simulink model "QuadrotorModel"  (R2023b)
settings: Solver=VariableStepAuto  StartTime=0.0  StopTime=120  RelTol=1e-3
undefined symbols (not defined in the file): A, a1, a2, a3, a4, a5, B, b1, b2, b3, belokan, C, c1, c2, c3, c4, c5, c6, c7, c8, D, g, k1, k2, k3, k4, kecepatan, kf, km, lebar, m, OM_r, panjang, phi_dot_d, psi_dot_d, theta_dot_d, U1, U1_max, U2, U2_max, U3, U4, U4_max, z_dot_d
libraries: simulink_extras x6, sldrtlib x1
settings Model: Creator=izmah  LastModifiedBy=izmah
settings SolverCC: ZeroCrossAlgorithm=Adaptive
settings DebuggingCC: IgnoredZcDiagnostic=none

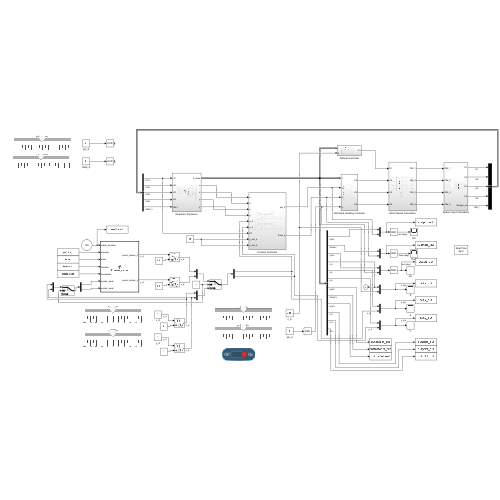
[thumbnail: Simulink's stored preview of the top-level diagram]
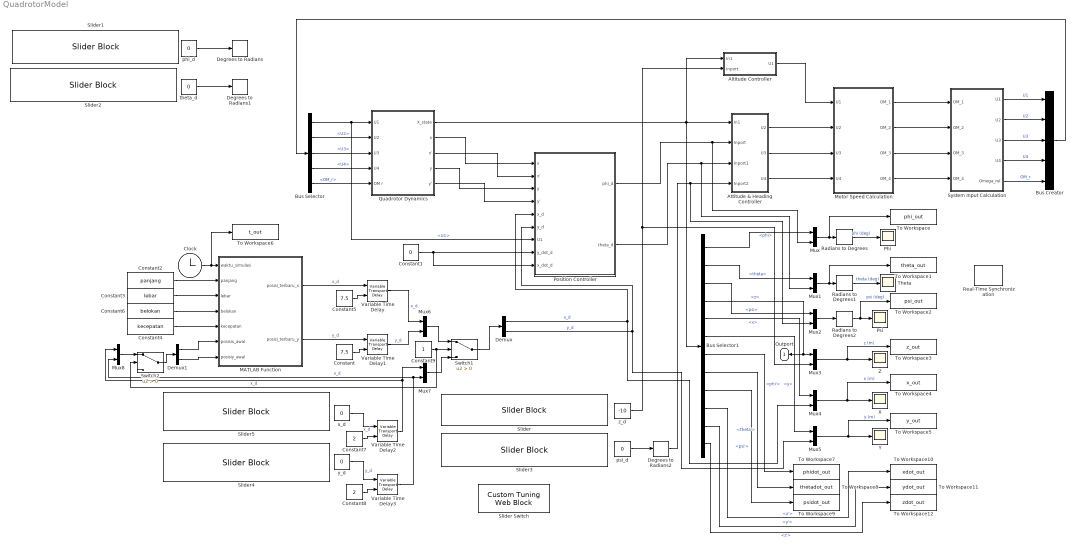
== system QuadrotorModel ==
  Altitude Controller : Subsystem
  Attitude & Heading Controller : Subsystem
  Bus Creator : BusCreator  Inputs=U1,U2,U3,U4,OM_r
  Bus Selector : BusSelector  OutputSignals=U1,U2,U3,U4,OM_r
  Bus Selector1 : BusSelector  OutputSignals=phi,theta,psi,z,x,y,phi',theta',psi',x',y',z'
  Clock : Clock
      settings: Decimation=waktu_simulasi
  Constant : Constant  Value=7.5
  Constant1 : Constant  Value=0
  Constant2 : Constant  Value=panjang
  Constant3 : Constant  Value=lebar
  Constant4 : Constant  Value=kecepatan
  Constant5 : Constant  Value=7.5
  Constant6 : Constant  Value=belokan
  Constant7 : Constant  Value=2
  Constant8 : Constant  Value=2
  Constant9 : Constant
  Degrees to Radians : simulink_extras/Transformations/Degrees to Radians
  Degrees to Radians1 : simulink_extras/Transformations/Degrees to Radians
  Degrees to Radians2 : simulink_extras/Transformations/Degrees to Radians
  Demux : Demux  Outputs=2
  Demux1 : Demux  Outputs=2
  MATLAB Function : MATLAB Function  TreatAsAtomicUnit=on
  Motor Speed Calculation : Subsystem
  Mux{,1..8} (9 alike) : Mux  Inputs=2
  Phi : Scope
  Position Controller : Subsystem
  Psi : Scope
  Quadrotor Dynamics : Subsystem
  Radians to Degrees : simulink_extras/Transformations/Radians to Degrees
  Radians to Degrees1 : simulink_extras/Transformations/Radians to Degrees
  Radians to Degrees2 : simulink_extras/Transformations/Radians to Degrees
  Real-Time Synchronization : sldrtlib/Real-Time Synchronization  SampleTime=0.1  MaxMissedTicks=1000  ShowMissedTicks=off  YieldWhenWaiting=off
  Slider : SliderBlock  ScaleMin=-20  ScaleMax=0
  Slider Switch : CustomTuningWebBlock  LabelPosition=Hide  ShowInitialText=on  Configuration="{\"components\":[{\"name\":\"CustomSwitchStateComponent\",\"settings\":{\"position\":[0,0,1,1],\"states\":[{\"HitRegion\":{\"position\":[0,0,0.5,1]},\"Image\":{\"position\":[0,0,1,1],\"size\":[1,1],\"src\":\"data:image\\/svg+xml;base64,PD94bWwgdmVyc2lvbj0iMS4wIiBlbmNvZGluZz0idXRmLTgiPz4NCjwhLS0gR2VuZXJhdG9yOiBBZG9iZSBJbGx1c3RyYXRvciAyNS4yLjEsIFNWRyBFeHBvcnQgUGx1Zy1JbiAuIFNWRyBWZXJzaW9uOiA2LjAwIEJ1aWxkIDApICAtLT4NCjxzdmcgdmVyc2lvbj0iMS4xIiB4bWxucz0iaHR0cDovL3d3dy53My5vcmcvMjAwMC9zdmciIHhtbG5zOnhsaW5rPSJodHRwOi8vd3d3LnczLm9yZy8xOTk5L3hsaW5rIiB4PSIwcHgiIHk9IjBweCINCgkgdmlld0JveD0iMCAwIDc2IDI5IiBzdHlsZT0iZW5hYmxlLWJhY2tncm91bmQ6bmV3 ...(+5404 chars)\",\"srcOrientation\":\"Right\"},\"Label\":{\"color\":[0.9882352941176471,0.9882352941176471,0.7725490196078432],\"icon\":{\"size\":[0,0],\"src\":[],\"srcOrientation\":\"Right\"},\"iconPlacement\":\"left\",\"opacity\":1,\"position\":[0.5,0.14],\"show\":true,\"text\":{\"content\":\"Off\",\"font\":\"Helvetica\",\"fontSize\":8.4}},\"Value\":-1},{\"HitRegion\":{\"position\":[0,0.5,0.5,1]},\"Image\":{\"position\":[0,0,1,1],\"size\":[1,1],\"src\":\"data:image\\/svg+xml;base64,PD94bWwgdmVyc2lvbj0iMS4wIiBlbmNvZGluZz0idXRmLTgiPz4NCjwhLS0gR2VuZXJhdG9yOiBBZG9iZSBJbGx1c3RyYXRvciAyNS4yLjEsIFNWRyBFeHBvcnQgUGx1Zy1JbiAuIFNWRyBWZXJzaW9uOiA2LjAwIEJ1aWxkIDApICAtLT4NCjxzdmcgdmVyc2lvbj0iMS4xIiB4bWxucz0iaHR0cDovL3d3dy53My5vcmcvMjAwMC9zdmciIHhtbG5zOnhsaW5rPSJodHRwOi8vd3d3LnczLm9yZy8xOTk5L3hsaW5rIiB4PSIwcHgiIHk9IjBweCINCgkgdmlld0JveD0iMCAwIDc2IDI5IiBzdHlsZT0iZW5hYmxlLWJhY2tncm91bmQ6bmV3 ...(+5404 chars)\",\"srcOrientation\":\"Right\"},\"Label\":{\"color\":[0.9882352941176471,0.9882352941176471,0.7725490196078432],\"icon\":{\"size\":[0,0],\"src\":[],\"srcOrientation\":\"Right\"},\"iconPlacement\":\"left\",\"opacity\":1,\"position\":[0.5,0.86],\"show\":true,\"text\":{\"content\":\"On\",\"font\":\"Helvetica\",\"fontSize\":8.4}},\"Value\":1}]}},{\"name\":\"BackgroundImageComponent\",\"settings\":{\"image\":{\"size\":[140,55],\"src\":\"default\",\"srcOrientation\":\"Right\"},\"position\":[0,0,1,1],\"scaleMode\":\"0\"}},{\"name\":\"ForegroundImageComponent\",\"settings\":{\"image\":{\"size\":[0,0],\"src\":\"default\",\"srcOrientation\":[]},\"isForeground\":1,\"position\":[0,0,1,1],\"scaleMode\":\"0\"}}],\"settings\":{\"BindingType\":\"param\",\"backgroundColor\":[0,0,255,\"1\"],\"backgroundOffset\":0.14,\"fixedAspectRatio\":\"on\",\"foregroundColor\":[234,234,234],\"showBackgroundColor\":false,\"variant\":\"slider\",\"version\":\"R2023a\"},\"type\":\"Switch\"}"
  Slider1 : SliderBlock  ScaleMin=-5  ScaleMax=5
  Slider2 : SliderBlock  ScaleMin=-5  ScaleMax=5
  Slider3 : SliderBlock  ScaleMin=-5  ScaleMax=5
  Slider4 : SliderBlock  ScaleMin=-20  ScaleMax=20
  Slider5 : SliderBlock  ScaleMin=-20  ScaleMax=20
  Switch1 : Switch  Criteria=u2 > Threshold  SaturateOnIntegerOverflow=off  InputSameDT=off
  Switch2 : Switch  Criteria=u2 > Threshold  SaturateOnIntegerOverflow=off  InputSameDT=off
  System Input Calculation : Subsystem
  Theta : Scope
  To Workspace : ToWorkspace  VariableName=phi_out  SaveFormat=Timeseries  SampleTime=-1
  To Workspace1 : ToWorkspace  VariableName=theta_out  SaveFormat=Timeseries  SampleTime=-1
  To Workspace10 : ToWorkspace  VariableName=xdot_out  SaveFormat=Timeseries  SampleTime=-1
  To Workspace11 : ToWorkspace  VariableName=ydot_out  SaveFormat=Timeseries  SampleTime=-1
  To Workspace12 : ToWorkspace  VariableName=zdot_out  SaveFormat=Timeseries  SampleTime=-1
  To Workspace2 : ToWorkspace  VariableName=psi_out  SaveFormat=Timeseries  SampleTime=-1
  To Workspace3 : ToWorkspace  VariableName=z_out  SaveFormat=Timeseries  SampleTime=-1
  To Workspace4 : ToWorkspace  VariableName=x_out  SaveFormat=Timeseries  SampleTime=-1
  To Workspace5 : ToWorkspace  VariableName=y_out  SaveFormat=Timeseries  SampleTime=-1
  To Workspace6 : ToWorkspace  VariableName=t_out  SaveFormat=Timeseries  SampleTime=-1
  To Workspace7 : ToWorkspace  VariableName=phidot_out  SaveFormat=Timeseries  SampleTime=-1
  To Workspace8 : ToWorkspace  VariableName=thetadot_out  SaveFormat=Timeseries  SampleTime=-1
  To Workspace9 : ToWorkspace  VariableName=psidot_out  SaveFormat=Timeseries  SampleTime=-1
  Variable Time Delay{,1..3} (4 alike) : VariableTransportDelay  MaximumDelay=10
  X : Scope
  Y : Scope
  Z : Scope
  phi_d : Constant  Value=0
  psi_d : Constant  Value=0
  theta_d : Constant  Value=0
  x_d : Constant  Value=0
  y_d : Constant  Value=0
  z_d : Constant  Value=-10
  Outport : Outport
  wires:
  Quadrotor Dynamics/1(X_state) -> Bus Selector1/1, Attitude & Heading Controller/1(In1), Altitude Controller/1(In1)
  Altitude Controller/1(U1) -> Motor Speed Calculation/1(U1)
  Attitude & Heading Controller/1(U2) -> Motor Speed Calculation/2(U2)
  Attitude & Heading Controller/2(U3) -> Motor Speed Calculation/3(U3)
  Attitude & Heading Controller/3(U4) -> Motor Speed Calculation/4(U4)
  Motor Speed Calculation/1(OM_1) -> System Input Calculation/1(OM_1)
  Motor Speed Calculation/2(OM_2) -> System Input Calculation/2(OM_2)
  Motor Speed Calculation/3(OM_3) -> System Input Calculation/3(OM_3)
  Motor Speed Calculation/4(OM_4) -> System Input Calculation/4(OM_4)
  System Input Calculation/1(U1) -> Bus Creator/1  "U1"
  System Input Calculation/2(U2) -> Bus Creator/2  "U2"
  System Input Calculation/3(U3) -> Bus Creator/3  "U3"
  System Input Calculation/4(U4) -> Bus Creator/4  "U4"
  System Input Calculation/5(Omega_rel) -> Bus Creator/5  "OM_r"
  Bus Creator/1 -> Bus Selector/1
  Mux/1 -> To Workspace/1, Radians to Degrees/1
  Radians to Degrees/1 -> Phi/1  "phi (deg)"
  Radians to Degrees1/1 -> Theta/1  "theta (deg)"
  Radians to Degrees2/1 -> Psi/1, To Workspace2/1  "psi (deg)"
  Bus Selector/1 -> Quadrotor Dynamics/1(U1), Position Controller/7(U1)  "<U1>"
  Bus Selector/2 -> Quadrotor Dynamics/2(U2)  "<U2>"
  Bus Selector/3 -> Quadrotor Dynamics/3(U3)  "<U3>"
  Bus Selector/4 -> Quadrotor Dynamics/4(U4)  "<U4>"
  Bus Selector/5 -> Quadrotor Dynamics/5(OM r)  "<OM_r>"
  Bus Selector1/1 -> Mux/1  "<phi>"
  Bus Selector1/2 -> Mux1/1  "<theta>"
  Mux1/1 -> To Workspace1/1, Radians to Degrees1/1
  Bus Selector1/3 -> Mux2/1  "<psi>"
  Mux2/1 -> Radians to Degrees2/1
  Bus Selector1/4 -> Mux3/1, Outport/1  "<z>"
  Mux3/1 -> Z/1, To Workspace3/1  "z (m)"
  z_d/1 -> Altitude Controller/2(Inport), Mux3/2
  phi_d/1 -> Degrees to Radians/1
  theta_d/1 -> Degrees to Radians1/1
  psi_d/1 -> Degrees to Radians2/1
  Quadrotor Dynamics/2(x) -> Position Controller/1(x)
  Quadrotor Dynamics/3(x') -> Position Controller/2(x')
  Quadrotor Dynamics/4(y) -> Position Controller/3(y)
  Quadrotor Dynamics/5(y') -> Position Controller/4(y')
  Degrees to Radians2/1 -> Mux2/2, Attitude & Heading Controller/4(Inport2)
  Position Controller/1(phi_d) -> Attitude & Heading Controller/2(Inport), Mux/2
  Position Controller/2(theta_d) -> Mux1/2, Attitude & Heading Controller/3(Inport1)
  Bus Selector1/5 -> Mux4/1  "<x>"
  Mux4/1 -> X/1, To Workspace4/1  "x (m)"
  Bus Selector1/6 -> Mux5/1  "<y>"
  Mux5/1 -> Y/1, To Workspace5/1  "y (m)"
  Constant1/1 -> Position Controller/8(y_dot_d), Position Controller/9(x_dot_d)
  Demux/1 -> Mux4/2, Position Controller/5(x_d)  "x_d"
  Demux/2 -> Mux5/2, Position Controller/6(y_d)  "y_d"
  Clock/1 -> To Workspace6/1, MATLAB Function/1(waktu_simulasi)
  Constant3/1 -> MATLAB Function/3(lebar)
  Constant2/1 -> MATLAB Function/2(panjang)
  Constant6/1 -> MATLAB Function/4(belokan)
  Constant4/1 -> MATLAB Function/5(kecepatan)
  MATLAB Function/1(posisi_terbaru_x) -> Variable Time Delay/1  "x_d"
  MATLAB Function/2(posisi_terbaru_y) -> Variable Time Delay1/1  "y_d"
  Constant5/1 -> Variable Time Delay/2
  Constant/1 -> Variable Time Delay1/2
  Variable Time Delay/1 -> Mux6/1  "x_d"
  Variable Time Delay1/1 -> Mux6/2  "y_d"
  Mux6/1 -> Switch1/1
  Switch1/1 -> Demux/1
  Mux7/1 -> Switch1/3
  Constant7/1 -> Variable Time Delay2/2
  Constant8/1 -> Variable Time Delay3/2
  x_d/1 -> Variable Time Delay2/1  "x_d"
  Variable Time Delay2/1 -> Mux7/1, Mux8/1  "x_d"
  y_d/1 -> Variable Time Delay3/1  "y_d"
  Variable Time Delay3/1 -> Mux8/2, Mux7/2  "x_d"
  Constant9/1 -> Switch1/2, Switch2/2
  Mux8/1 -> Switch2/1
  Switch2/1 -> Demux1/1
  Demux1/1 -> MATLAB Function/6(posisix_awal)
  Demux1/2 -> MATLAB Function/7(posisiy_awal)
  Bus Selector1/7 -> To Workspace7/1  "<phi'>"
  Bus Selector1/8 -> To Workspace8/1  "<theta'>"
  Bus Selector1/9 -> To Workspace9/1  "<psi'>"
  Bus Selector1/10 -> To Workspace10/1  "<x'>"
  Bus Selector1/11 -> To Workspace11/1  "<y'>"
  Bus Selector1/12 -> To Workspace12/1  "<z'>"

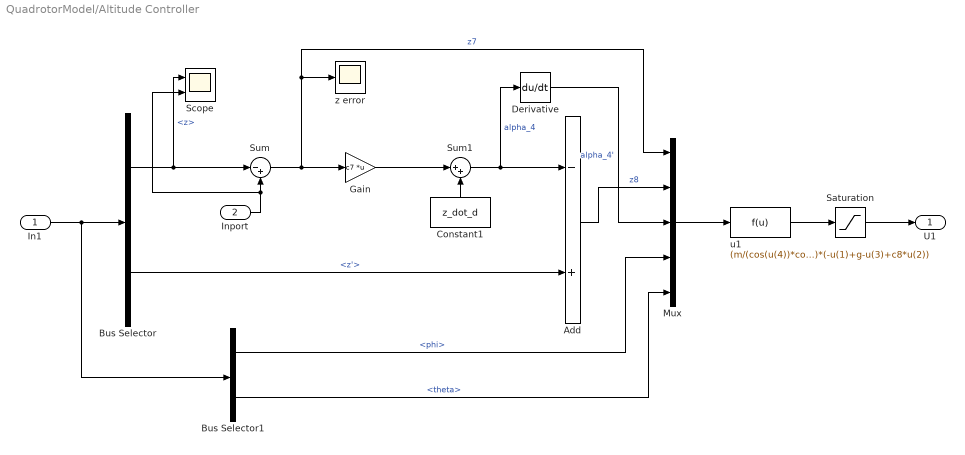
== system QuadrotorModel/Altitude Controller ==
  In1 : Inport
  Inport : Inport  Port=2
  Add : Sum  Inputs=-+
  Bus Selector : BusSelector  OutputSignals=z,z'
  Bus Selector1 : BusSelector  OutputSignals=phi,theta
  Constant1 : Constant  Value=z_dot_d
  Derivative : Derivative
  Gain : Gain  Gain=c7  Multiplication=Matrix(K*u)
  Mux : Mux  Inputs=5
  Saturation : Saturate  UpperLimit=U1_max  LowerLimit=-inf
  Scope : Scope  NumInputPorts=2
  Sum : Sum  Inputs=|-+
  Sum1 : Sum  Inputs=|++
  u1 : Fcn  Expr=(m/(cos(u(4))*cos(u(5))))*(-u(1)+g-u(3)+c8*u(2))
  z error : Scope
  U1 : Outport
  wires:
  In1/1 -> Bus Selector/1, Bus Selector1/1
  Bus Selector/1 -> Scope/1, Sum/1  "<z>"
  Inport/1 -> Scope/2, Sum/2
  Sum/1 -> z error/1, Mux/1, Gain/1  "z7"
  Gain/1 -> Sum1/1
  Constant1/1 -> Sum1/2
  Sum1/1 -> Derivative/1, Add/1  "alpha_4"
  Bus Selector/2 -> Add/2  "<z'>"
  Derivative/1 -> Mux/3  "alpha_4'"
  Add/1 -> Mux/2  "z8"
  Bus Selector1/1 -> Mux/4  "<phi>"
  Bus Selector1/2 -> Mux/5  "<theta>"
  Mux/1 -> u1/1
  u1/1 -> Saturation/1
  Saturation/1 -> U1/1

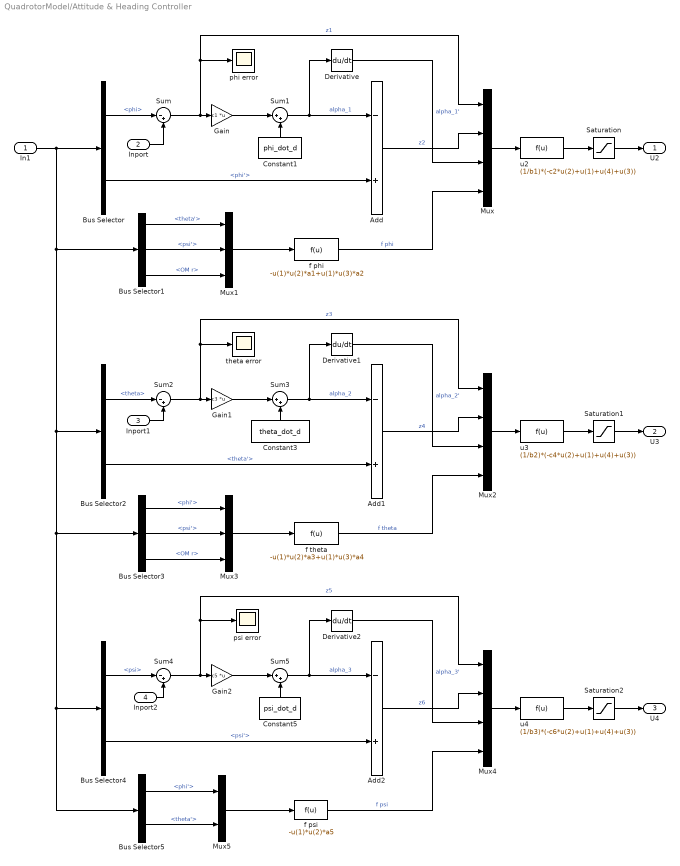
== system QuadrotorModel/Attitude & Heading Controller ==
  In1 : Inport
  Inport : Inport  Port=2
  Inport1 : Inport  Port=3
  Inport2 : Inport  Port=4
  Add : Sum  Inputs=-+
  Add1 : Sum  Inputs=-+
  Add2 : Sum  Inputs=-+
  Bus Selector : BusSelector  OutputSignals=phi,phi'
  Bus Selector1 : BusSelector  OutputSignals=theta',psi',OM r
  Bus Selector2 : BusSelector  OutputSignals=theta,theta'
  Bus Selector3 : BusSelector  OutputSignals=phi',psi',OM r
  Bus Selector4 : BusSelector  OutputSignals=psi,psi'
  Bus Selector5 : BusSelector  OutputSignals=phi',theta'
  Constant1 : Constant  Value=phi_dot_d
  Constant3 : Constant  Value=theta_dot_d
  Constant5 : Constant  Value=psi_dot_d
  Derivative : Derivative
  Derivative1 : Derivative
  Derivative2 : Derivative
  Gain : Gain  Gain=c1  Multiplication=Matrix(K*u)
  Gain1 : Gain  Gain=c3  Multiplication=Matrix(K*u)
  Gain2 : Gain  Gain=c5  Multiplication=Matrix(K*u)
  Mux : Mux
  Mux1 : Mux  Inputs=3
  Mux2 : Mux
  Mux3 : Mux  Inputs=3
  Mux4 : Mux
  Mux5 : Mux  Inputs=2
  Saturation : Saturate  UpperLimit=U2_max  LowerLimit=-inf
  Saturation1 : Saturate  UpperLimit=U2_max  LowerLimit=-inf
  Saturation2 : Saturate  UpperLimit=U4_max  LowerLimit=-inf
  Sum : Sum  Inputs=|-+
  Sum1 : Sum  Inputs=|++
  Sum2 : Sum  Inputs=|-+
  Sum3 : Sum  Inputs=|++
  Sum4 : Sum  Inputs=|-+
  Sum5 : Sum  Inputs=|++
  f phi : Fcn  Expr=-u(1)*u(2)*a1+u(1)*u(3)*a2
  f psi : Fcn  Expr=-u(1)*u(2)*a5
  f theta : Fcn  Expr=-u(1)*u(2)*a3+u(1)*u(3)*a4
  phi error : Scope
  psi error : Scope
  theta error : Scope
  u2 : Fcn  Expr=(1/b1)*(-c2*u(2)+u(1)+u(4)+u(3))
  u3 : Fcn  Expr=(1/b2)*(-c4*u(2)+u(1)+u(4)+u(3))
  u4 : Fcn  Expr=(1/b3)*(-c6*u(2)+u(1)+u(4)+u(3))
  U2 : Outport
  U3 : Outport  Port=2
  U4 : Outport  Port=3
  wires:
  Bus Selector/1 -> Sum/1  "<phi>"
  Inport/1 -> Sum/2
  Constant1/1 -> Sum1/2
  Sum1/1 -> Add/1, Derivative/1  "alpha_1"
  Bus Selector/2 -> Add/2  "<phi'>"
  Sum/1 -> phi error/1, Mux/1, Gain/1  "z1"
  Gain/1 -> Sum1/1
  Derivative/1 -> Mux/3  "alpha_1'"
  Add/1 -> Mux/2  "z2"
  Mux1/1 -> f phi/1
  f phi/1 -> Mux/4  "f phi"
  Mux/1 -> u2/1
  u2/1 -> Saturation/1
  u3/1 -> Saturation1/1
  Add1/1 -> Mux2/2  "z4"
  Sum3/1 -> Add1/1, Derivative1/1  "alpha_2"
  Mux3/1 -> f theta/1
  Constant3/1 -> Sum3/2
  Derivative1/1 -> Mux2/3  "alpha_2'"
  f theta/1 -> Mux2/4  "f theta"
  Sum2/1 -> Mux2/1, theta error/1, Gain1/1  "z3"
  Bus Selector2/1 -> Sum2/1  "<theta>"
  Gain1/1 -> Sum3/1
  Mux2/1 -> u3/1
  Bus Selector2/2 -> Add1/2  "<theta'>"
  u4/1 -> Saturation2/1
  Add2/1 -> Mux4/2  "z6"
  Sum5/1 -> Add2/1, Derivative2/1  "alpha_3"
  Mux5/1 -> f psi/1
  Constant5/1 -> Sum5/2
  Derivative2/1 -> Mux4/3  "alpha_3'"
  f psi/1 -> Mux4/4  "f psi"
  Sum4/1 -> psi error/1, Mux4/1, Gain2/1  "z5"
  In1/1 -> Bus Selector5/1, Bus Selector4/1, Bus Selector3/1, Bus Selector2/1, Bus Selector1/1, Bus Selector/1
  Bus Selector4/1 -> Sum4/1  "<psi>"
  Gain2/1 -> Sum5/1
  Mux4/1 -> u4/1
  Bus Selector4/2 -> Add2/2  "<psi'>"
  Bus Selector1/1 -> Mux1/1  "<theta'>"
  Bus Selector1/2 -> Mux1/2  "<psi'>"
  Bus Selector1/3 -> Mux1/3  "<OM r>"
  Bus Selector3/1 -> Mux3/1  "<phi'>"
  Bus Selector3/2 -> Mux3/2  "<psi'>"
  Bus Selector3/3 -> Mux3/3  "<OM r>"
  Bus Selector5/1 -> Mux5/1  "<phi'>"
  Bus Selector5/2 -> Mux5/2  "<theta'>"
  Saturation/1 -> U2/1
  Saturation1/1 -> U3/1
  Saturation2/1 -> U4/1
  Inport1/1 -> Sum2/2
  Inport2/1 -> Sum4/2

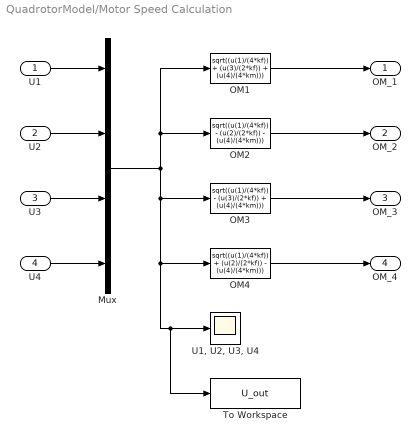
== system QuadrotorModel/Motor Speed Calculation ==
  U1 : Inport
  U2 : Inport  Port=2
  U3 : Inport  Port=3
  U4 : Inport  Port=4
  Mux : Mux
  OM1 : Fcn  Expr=sqrt((u(1)/(4*kf)) + (u(3)/(2*kf)) + (u(4)/(4*km)))
  OM2 : Fcn  Expr=sqrt((u(1)/(4*kf)) - (u(2)/(2*kf)) - (u(4)/(4*km)))
  OM3 : Fcn  Expr=sqrt((u(1)/(4*kf)) - (u(3)/(2*kf)) + (u(4)/(4*km)))
  OM4 : Fcn  Expr=sqrt((u(1)/(4*kf)) + (u(2)/(2*kf)) - (u(4)/(4*km)))
  To Workspace : ToWorkspace  VariableName=U_out  SaveFormat=Timeseries  SampleTime=-1
  "U1, U2, U3, U4" : Scope
  OM_1 : Outport
  OM_2 : Outport  Port=2
  OM_3 : Outport  Port=3
  OM_4 : Outport  Port=4
  wires:
  U1/1 -> Mux/1
  U2/1 -> Mux/2
  U3/1 -> Mux/3
  U4/1 -> Mux/4
  OM1/1 -> OM_1/1
  OM2/1 -> OM_2/1
  OM3/1 -> OM_3/1
  OM4/1 -> OM_4/1
  Mux/1 -> "U1, U2, U3, U4"/1, To Workspace/1, OM4/1, OM3/1, OM2/1, OM1/1

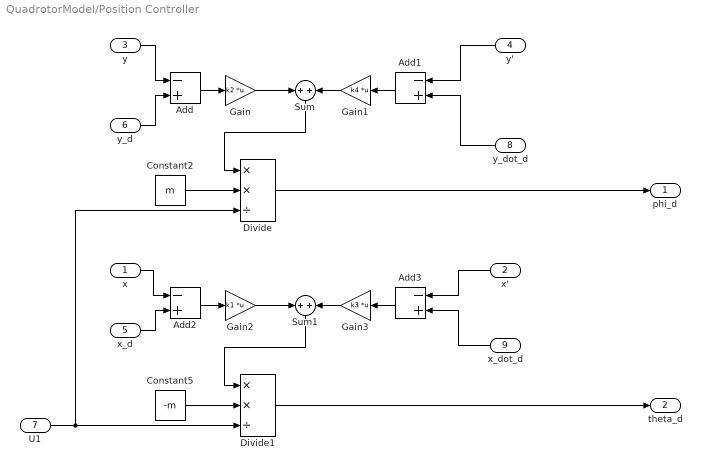
== system QuadrotorModel/Position Controller ==
  x : Inport
  x' : Inport  Port=2
  y : Inport  Port=3
  y' : Inport  Port=4
  x_d : Inport  Port=5
  y_d : Inport  Port=6
  U1 : Inport  Port=7
  y_dot_d : Inport  Port=8
  x_dot_d : Inport  Port=9
  Add{,1..3} (4 alike) : Sum  Inputs=-+
  Constant2 : Constant  Value=m
  Constant5 : Constant  Value=-m
  Divide : Product  Inputs=**/
  Divide1 : Product  Inputs=**/
  Gain : Gain  Gain=k2  Multiplication=Matrix(K*u)
  Gain1 : Gain  Gain=k4  Multiplication=Matrix(K*u)
  Gain2 : Gain  Gain=k1  Multiplication=Matrix(K*u)
  Gain3 : Gain  Gain=k3  Multiplication=Matrix(K*u)
  Sum : Sum  Inputs=+|+
  Sum1 : Sum  Inputs=+|+
  phi_d : Outport
  theta_d : Outport  Port=2
  wires:
  Gain3/1 -> Sum1/2
  Add2/1 -> Gain2/1
  Add3/1 -> Gain3/1
  Sum1/1 -> Divide1/1
  x_dot_d/1 -> Add3/2
  Gain2/1 -> Sum1/1
  Constant5/1 -> Divide1/2
  Constant2/1 -> Divide/2
  Gain/1 -> Sum/1
  Gain1/1 -> Sum/2
  Sum/1 -> Divide/1
  y_dot_d/1 -> Add1/2
  Add1/1 -> Gain1/1
  Add/1 -> Gain/1
  x_d/1 -> Add2/2
  y_d/1 -> Add/2
  Divide/1 -> phi_d/1
  Divide1/1 -> theta_d/1
  x/1 -> Add2/1
  x'/1 -> Add3/1
  y/1 -> Add/1
  y'/1 -> Add1/1
  U1/1 -> Divide/3, Divide1/3

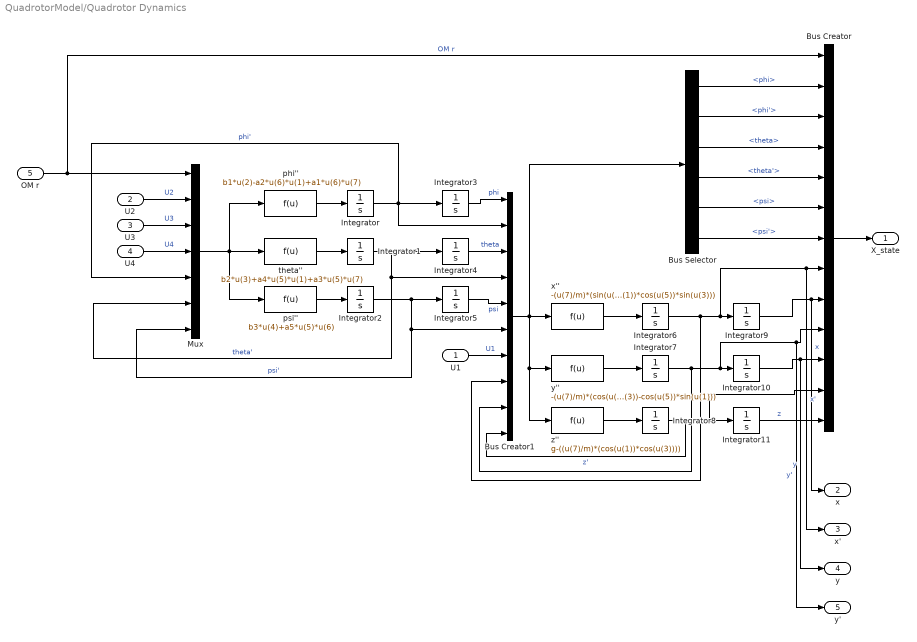
== system QuadrotorModel/Quadrotor Dynamics ==
  U1 : Inport
  U2 : Inport  Port=2
  U3 : Inport  Port=3
  U4 : Inport  Port=4
  OM r : Inport  Port=5
  Bus Creator : BusCreator  Inputs=13
  Bus Creator1 : BusCreator  Inputs=10
  Bus Selector : BusSelector  OutputSignals=phi,phi',theta,theta',psi,psi'
  Integrator{,1..11} (12 alike) : Integrator
  Mux : Mux  Inputs=7
  phi'' : Fcn  Expr=b1*u(2)-a2*u(6)*u(1)+a1*u(6)*u(7)
  psi'' : Fcn  Expr=b3*u(4)+a5*u(5)*u(6)
  theta'' : Fcn  Expr=b2*u(3)+a4*u(5)*u(1)+a3*u(5)*u(7)
  x'' : Fcn  Expr=-(u(7)/m)*(sin(u(1))*sin(u(5))+cos(u(1))*cos(u(5))*sin(u(3)))
  y'' : Fcn  Expr=-(u(7)/m)*(cos(u(1))*sin(u(5))*sin(u(3))-cos(u(5))*sin(u(1)))
  z'' : Fcn  Expr=g-((u(7)/m)*(cos(u(1))*cos(u(3))))
  X_state : Outport
  x : Outport  Port=2
  x' : Outport  Port=3
  y : Outport  Port=4
  y' : Outport  Port=5
  wires:
  Bus Creator/1 -> X_state/1
  U2/1 -> Mux/2  "U2"
  U3/1 -> Mux/3  "U3"
  U4/1 -> Mux/4  "U4"
  OM r/1 -> Mux/1, Bus Creator/1  "OM r"
  Mux/1 -> psi''/1, phi''/1, theta''/1
  phi''/1 -> Integrator/1
  theta''/1 -> Integrator1/1
  psi''/1 -> Integrator2/1
  Integrator/1 -> Mux/5, Integrator3/1, Bus Creator1/2  "phi'"
  Integrator1/1 -> Integrator4/1, Mux/6, Bus Creator1/4  "theta'"
  Integrator2/1 -> Bus Creator1/6, Mux/7, Integrator5/1  "psi'"
  Integrator3/1 -> Bus Creator1/1  "phi"
  Integrator4/1 -> Bus Creator1/3  "theta"
  Integrator5/1 -> Bus Creator1/5  "psi"
  U1/1 -> Bus Creator1/7  "U1"
  x''/1 -> Integrator6/1
  y''/1 -> Integrator7/1
  z''/1 -> Integrator8/1
  Integrator6/1 -> Bus Creator1/8, x'/1, Bus Creator/8, Integrator9/1  "x'"
  Integrator7/1 -> Bus Creator1/9, Bus Creator/10, y'/1, Integrator10/1  "y'"
  Integrator8/1 -> Bus Creator/12, Integrator11/1, Bus Creator1/10  "z'"
  Integrator11/1 -> Bus Creator/13  "z"
  Integrator10/1 -> y/1, Bus Creator/11  "y"
  Integrator9/1 -> x/1, Bus Creator/9  "x"
  Bus Creator1/1 -> Bus Selector/1, x''/1, z''/1, y''/1
  Bus Selector/4 -> Bus Creator/5  "<theta'>"
  Bus Selector/1 -> Bus Creator/2  "<phi>"
  Bus Selector/2 -> Bus Creator/3  "<phi'>"
  Bus Selector/3 -> Bus Creator/4  "<theta>"
  Bus Selector/5 -> Bus Creator/6  "<psi>"
  Bus Selector/6 -> Bus Creator/7  "<psi'>"

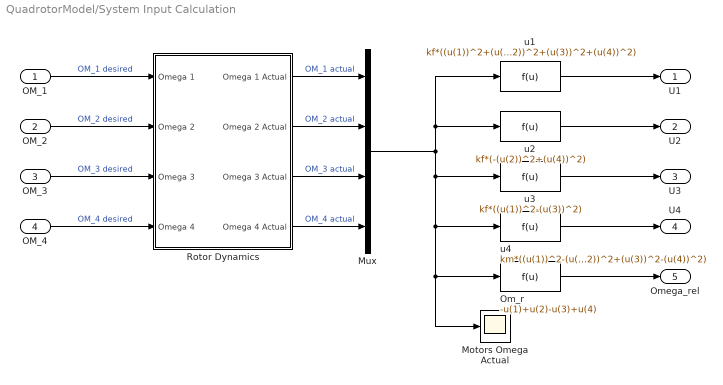
== system QuadrotorModel/System Input Calculation ==
  OM_1 : Inport
  OM_2 : Inport  Port=2
  OM_3 : Inport  Port=3
  OM_4 : Inport  Port=4
  Motors Omega Actual : Scope
  Mux : Mux
  Om_r : Fcn  Expr=-u(1)+u(2)-u(3)+u(4)
  Rotor Dynamics : Subsystem
  u1 : Fcn  Expr=kf*((u(1))^2+(u(2))^2+(u(3))^2+(u(4))^2)
  u2 : Fcn  Expr=kf*(-(u(2))^2+(u(4))^2)
  u3 : Fcn  Expr=kf*((u(1))^2-(u(3))^2)
  u4 : Fcn  Expr=km*((u(1))^2-(u(2))^2+(u(3))^2-(u(4))^2)
  U1 : Outport
  U2 : Outport  Port=2
  U3 : Outport  Port=3
  U4 : Outport  Port=4
  Omega_rel : Outport  Port=5
  wires:
  OM_1/1 -> Rotor Dynamics/1(Omega 1)  "OM_1 desired"
  OM_2/1 -> Rotor Dynamics/2(Omega 2)  "OM_2 desired"
  OM_3/1 -> Rotor Dynamics/3(Omega 3)  "OM_3 desired"
  OM_4/1 -> Rotor Dynamics/4(Omega 4)  "OM_4 desired"
  Rotor Dynamics/1(Omega 1 Actual) -> Mux/1  "OM_1 actual"
  Rotor Dynamics/2(Omega 2 Actual) -> Mux/2  "OM_2 actual"
  Rotor Dynamics/3(Omega 3 Actual) -> Mux/3  "OM_3 actual"
  Rotor Dynamics/4(Omega 4 Actual) -> Mux/4  "OM_4 actual"
  u1/1 -> U1/1
  u2/1 -> U2/1
  u3/1 -> U3/1
  u4/1 -> U4/1
  Om_r/1 -> Omega_rel/1
  Mux/1 -> Motors Omega Actual/1, Om_r/1, u4/1, u3/1, u2/1, u1/1

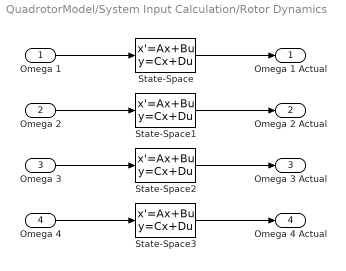
== system QuadrotorModel/System Input Calculation/Rotor Dynamics ==
  Omega 1 : Inport
  Omega 2 : Inport  Port=2
  Omega 3 : Inport  Port=3
  Omega 4 : Inport  Port=4
  State-Space{,1..3} (4 alike) : StateSpace  A=A  B=B  C=C  D=D  InitialCondition=0.01
  Omega 1 Actual : Outport
  Omega 2 Actual : Outport  Port=2
  Omega 3 Actual : Outport  Port=3
  Omega 4 Actual : Outport  Port=4
  wires:
  Omega 4/1 -> State-Space3/1
  Omega 3/1 -> State-Space2/1
  Omega 2/1 -> State-Space1/1
  Omega 1/1 -> State-Space/1
  State-Space/1 -> Omega 1 Actual/1
  State-Space1/1 -> Omega 2 Actual/1
  State-Space2/1 -> Omega 3 Actual/1
  State-Space3/1 -> Omega 4 Actual/1

== matlab function QuadrotorModel/MATLAB Function ==
  data: waktu_simulasi input; panjang input; lebar input; belokan input; kecepatan input; posisi_terbaru_x output; posisi_terbaru_y output; posisix_awal input; posisiy_awal input
% Fungsi untuk menghasilkan lintasan drone zig-zag
function [posisi_terbaru_x, posisi_terbaru_y] = lintasan_drone( waktu_simulasi, panjang, lebar, belokan, kecepatan, posisix_awal, posisiy_awal)
    % Inisialisasi
    posisi_terbaru_x = posisix_awal;
    posisi_terbaru_y = posisiy_awal;

    % Jumlah lintasan pada sumbu y
    jumlah_belokan = ceil(lebar / belokan);

    % Inisialisasi lintasan
    x_d = posisix_awal;
    y_d = posisiy_awal;
    waktu_d = 0; % Waktu untuk setiap titik lintasan

    % Variabel posisi awal
    x_pos = posisix_awal;
    y_pos = posisiy_awal;
    arah_x = 1; % 1: ke kanan, -1: ke kiri
    waktu_total = 0; % Waktu total lintasan

    % Iterasi untuk membuat lintasan zig-zag
    for i = 1:jumlah_belokan
        % Tentukan arah gerakan pada sumbu x (ke kanan atau ke kiri)
        x_target = x_pos + arah_x * panjang;

        % Buat lintasan pada sumbu x
        t_x = abs(x_target - x_pos) / kecepatan; % waktu tempuh pada x
        t_segment = linspace(waktu_total, waktu_total + t_x, 100);
        x_segment = linspace(x_pos, x_target, 100);
        y_segment = y_pos * ones(size(x_segment));

        % Tambahkan ke lintasan
        x_d = [x_d, x_segment];
        y_d = [y_d, y_segment];
        waktu_d = [waktu_d, t_segment];

        % Perbarui posisi x dan waktu total
        x_pos = x_target;
        waktu_total = waktu_total + t_x;

        % Tentukan posisi y untuk belokan berikutnya
        if i < jumlah_belokan
            y_target = y_pos + belokan;
            t_y = belokan / kecepatan; % waktu tempuh pada y
            t_segment = linspace(waktu_total, waktu_total + t_y, 100);
            x_segment = x_pos * ones(size(t_segment));
            y_segment = linspace(y_pos, y_target, 100);

            % Tambahkan ke lintasan
            x_d = [x_d, x_segment];
            y_d = [y_d, y_segment];
            waktu_d = [waktu_d, t_segment];

            % Perbarui posisi y dan waktu total
            y_pos = y_target;
            waktu_total = waktu_total + t_y;

            % Ganti arah gerakan sumbu x
            arah_x = -arah_x; % Membalik arah (ke kiri atau ke kanan)
        end

        % Cek jika waktu simulasi sudah tercapai
        if waktu_total >= waktu_simulasi
            break;
        end
    end

    % Pastikan mencapai y paling ujung
    if y_pos < lebar + posisiy_awal && waktu_total < waktu_simulasi
        y_target = lebar + posisiy_awal;
        t_y = (y_target - y_pos) / kecepatan;
        t_segment = linspace(waktu_total, waktu_total + t_y, 100);
        x_segment = x_pos * ones(size(t_segment));
        y_segment = linspace(y_pos, y_target, 100);

        % Tambahkan ke lintasan
        x_d = [x_d, x_segment];
        y_d = [y_d, y_segment];
        waktu_d = [waktu_d, t_segment];

        % Perbarui posisi y dan waktu total
        y_pos = y_target;
        waktu_total = waktu_total + t_y;

        % Perbarui arah lintasan sumbu x agar drone terus bergerak
        arah_x = -1 * arah_x; % Membalik arah x agar terus zig-zag
        x_target = x_pos + arah_x * panjang;

        % Buat lintasan pada sumbu x setelah mencapai y ujung
        t_x = abs(x_target - x_pos) / kecepatan; % waktu tempuh pada x
        t_segment = linspace(waktu_total, waktu_total + t_x, 100);
        x_segment = linspace(x_pos, x_target, 100);
        y_segment = y_pos * ones(size(x_segment));

        % Tambahkan lintasan baru
        x_d = [x_d, x_segment];
        y_d = [y_d, y_segment];
        waktu_d = [waktu_d, t_segment];

        % Perbarui posisi x
        x_pos = x_target;
        waktu_total = waktu_total + t_x;
    end

    % Kembali ke titik asal
    if x_pos == 0
        % Jika posisi terakhir di kiri (x = 0), hanya bergerak di sumbu y
        waktu_return = abs(y_pos - posisiy_awal) / kecepatan; % Menghitung waktu untuk kembali ke posisi awal y
        t_segment = linspace(waktu_total, waktu_total + waktu_return, 100);
        x_segment = posisix_awal * ones(size(t_segment)); % Tetap di x = posisix_awal
        y_segment = linspace(y_pos, posisiy_awal, 100); % Gerakan ke posisiy_awal
    else
        % Jika posisi terakhir di kanan (x ≠ 0), bergerak diagonal ke (posisix_awal, posisiy_awal)
        jarak = sqrt((x_pos - posisix_awal)^2 + (y_pos - posisiy_awal)^2); % Jarak diagonal ke titik asal
        waktu_return = jarak / kecepatan; % Waktu tempuh
        t_segment = linspace(waktu_total, waktu_total + waktu_return, 100);
        x_segment = linspace(x_pos, posisix_awal, 100); % Gerakan dari x_pos ke posisix_awal
        y_segment = linspace(y_pos, posisiy_awal, 100); % Gerakan dari y_pos ke posisiy_awal
    end

    % Tambahkan lintasan kembali ke titik asal
    x_d = [x_d, x_segment];
    y_d = [y_d, y_segment];
    waktu_d = [waktu_d, t_segment];

    % Perbarui waktu total
    waktu_total = waktu_total + waktu_return;

    % Jika waktu simulasi masih tersisa, tambahkan posisi diam di titik asal
    if waktu_total < waktu_simulasi
        waktu_diam = linspace(waktu_total, waktu_simulasi, 100);
        x_d = [x_d, posisix_awal * ones(size(waktu_diam))]; % Tetap di x = posisix_awal
        y_d = [y_d, posisiy_awal * ones(size(waktu_diam))]; % Tetap di y = posisiy_awal
        waktu_d = [waktu_d, waktu_diam];
    end


    % % Plot lintasan dengan animasi
    % figure;
    for k = 1:length(x_d)
        % % Plot lintasan dan posisi drone saat ini
        % plot(x_d(1:k), y_d(1:k), 'r', 'LineWidth', 1.5);
        % hold on;
        % plot(x_d(k), y_d(k), 'bo', 'MarkerFaceColor', 'b'); % Posisi drone saat ini
        % xlabel('Posisi x');
        % ylabel('Posisi y');
        % title('Lintasan Drone Zig-Zag');
        % grid on;
        % axis([min(x_d)-1, max(x_d)+1, min(y_d)-1, max(y_d)+1]);
        % hold off;

        % Ambil data posisi terbaru (1x1)
        posisi_terbaru_x = x_d(k);
        posisi_terbaru_y = y_d(k);

        % % Tampilkan posisi terbaru dan waktu ke Command Window
        % fprintf('Waktu: %.2f detik | Posisi terbaru: x = %.2f, y = %.2f\n', waktu_d(k), posisi_terbaru_x, posisi_terbaru_y);

        % % Pause untuk animasi
        % pause(0.01);

        % Hentikan animasi jika waktu simulasi habis
        if waktu_d(k) >= waktu_simulasi
            break;
        end
    end
end
